simulink model "SimulacaoMaquinaCCBlocoConstruido"  (R2022b)
settings: Solver=VariableStepAuto  StartTime=0.0  StopTime=10  MaxStep=1e-4  RelTol=1e-3
libraries: spspowerguiLib x1
settings Model: Creator=marcone.faria  LastModifiedBy=dedep
settings ModelReferenceCC: EnableRefExpFcnMdlSchedulingChecks=on

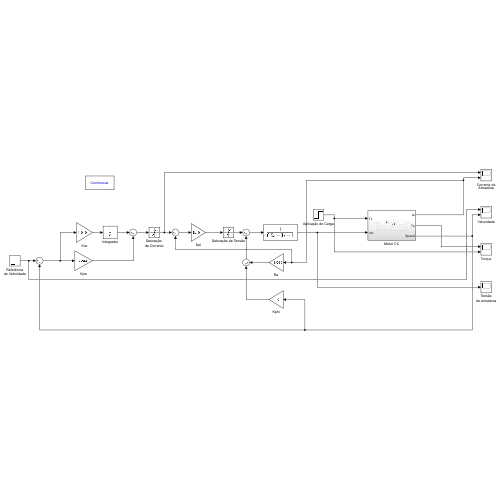
[thumbnail: Simulink's stored preview of the top-level diagram]
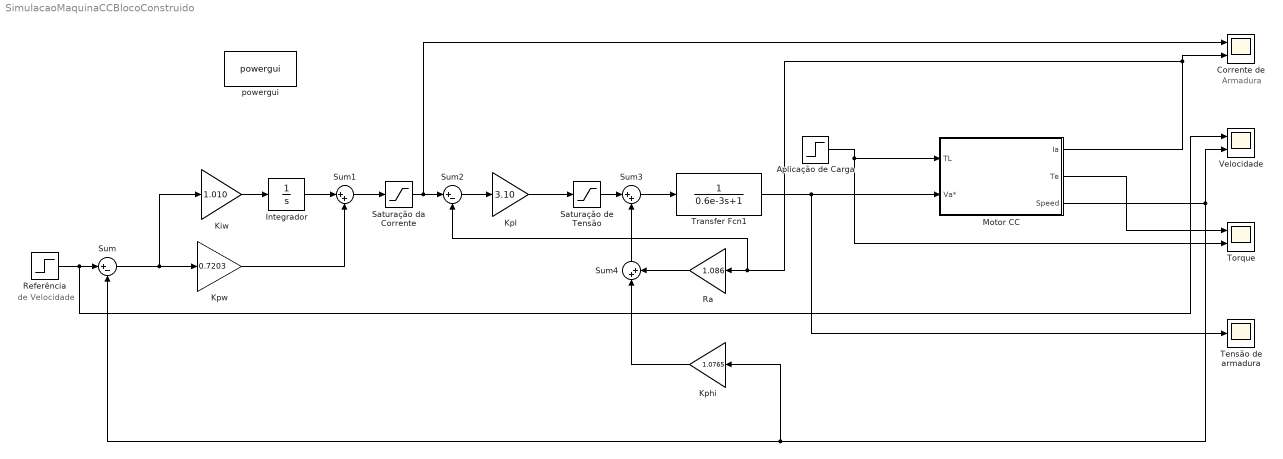
== system SimulacaoMaquinaCCBlocoConstruido ==
  note: Armadura
  note: de Velocidade
  Aplicação de Carga : Step  Before=20  After=40  SampleTime=0
  Corrente de : Scope  NumInputPorts=2
  Integrador : TransferFcn  Denominator=[1 0]
  Kiw : Gain  Gain=1.010
  Kphi : Gain  Gain=1.0765
  Kpl : Gain  Gain=3.10
  Kpw : Gain  Gain=0.7203
  Motor CC : Subsystem
  Ra : Gain  Gain=1.086
  Referência : Step  Time=0  After=92  SampleTime=0
  Saturação da Corrente : Saturate  UpperLimit=72  LowerLimit=-72
  Saturação de Tensão : Saturate  UpperLimit=360  LowerLimit=-360
  Sum : Sum  Inputs=|+-
  Sum1 : Sum  Inputs=|++
  Sum2 : Sum  Inputs=|+-
  Sum3 : Sum  Inputs=|++
  Sum4 : Sum  Inputs=|++
  Tensão de armadura : Scope
  Torque : Scope  NumInputPorts=2
  Transfer Fcn1 : TransferFcn  Denominator=[0.6e-3 1]
  Velocidade : Scope  NumInputPorts=2
  powergui : spspowerguiLib/powergui  Priority=1  SimulationMode=Continuous  SampleTime=50e-6  frequency=60  Iterations=50  frequencyindice=0  Pbase=100e6  ErrMax=1e-4  UnitsV=kV  UnitsW=MW  buscounter=0  FunctionMessages=off  echomessages=off  EnableUseOfTLC=off  CurrentSourceSwitches=off  DisableSnubberDevices=off  DisableRonSwitches=off  DisableVfSwitches=off  DisplayEquations=off  AutomaticDiscreteSolvers=off  SolverType=Tustin/Backward Euler (TBE)  Interpol=off  ExternalGateDelay=off  methode=off  Ts=100  x0status=blocks  SPID=on  SwTol=0  HookPort=off  NonlinearTolerance=1e-4  nMaxIteration=100  ContinueOnMaxIteration=off  RestoreLinks=warning  ResistiveCurrentMeasurement=off  Frange=[0:2:500]  Ylog=off  Xlog=on  ShowGrid=off  save=off  variable=ZData  structure=0  ZoomFFT=off  StartTime=0.0  cycles=1  DisplayStyle=1  fundamental=60  FreqAxis=off  MaxFrequency=1000  frequencyindicesteady=1  RmsSteady=1  display=off
  wires:
  Referência/1 -> Velocidade/1, Sum/1
  Sum/1 -> Kiw/1, Kpw/1
  Kiw/1 -> Integrador/1
  Integrador/1 -> Sum1/1
  Kpw/1 -> Sum1/2
  Sum1/1 -> Saturação da Corrente/1
  Saturação da Corrente/1 -> Corrente de/1, Sum2/1
  Sum2/1 -> Kpl/1
  Kpl/1 -> Saturação de Tensão/1
  Saturação de Tensão/1 -> Sum3/1
  Sum3/1 -> Transfer Fcn1/1
  Sum4/1 -> Sum3/2
  Ra/1 -> Sum4/2
  Kphi/1 -> Sum4/1
  Aplicação de Carga/1 -> Motor CC/1(TL), Torque/2
  Transfer Fcn1/1 -> Tensão de armadura/1, Motor CC/2(Va*)
  Motor CC/3(Speed) -> Velocidade/2, Kphi/1, Sum/2
  Motor CC/1(Ia) -> Corrente de/2, Sum2/2, Ra/1
  Motor CC/2(Te) -> Torque/1

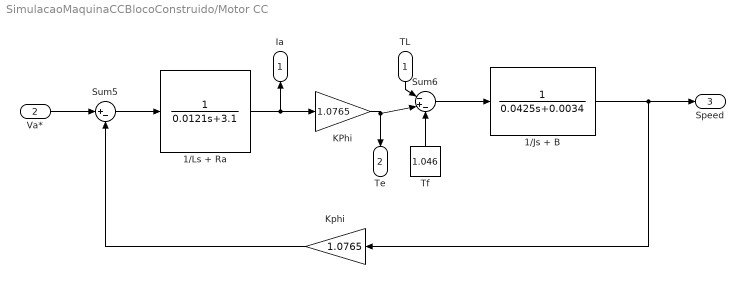
== system SimulacaoMaquinaCCBlocoConstruido/Motor CC ==
  TL : Inport
  Va* : Inport  Port=2
  1/Js + B : TransferFcn  Denominator=[0.0425 0.0034]
  1/Ls + Ra : TransferFcn  Denominator=[0.0121 3.1]
  KPhi : Gain  Gain=1.0765
  Kphi : Gain  Gain=1.0765
  Sum5 : Sum  Inputs=|+-
  Sum6 : Sum  Inputs=|-+-
  Tf : Constant  Value=1.046
  Ia : Outport
  Te : Outport  Port=2
  Speed : Outport  Port=3
  wires:
  1/Js + B/1 -> Kphi/1, Speed/1
  KPhi/1 -> Sum6/2, Te/1
  Tf/1 -> Sum6/3
  Sum5/1 -> 1/Ls + Ra/1
  1/Ls + Ra/1 -> KPhi/1, Ia/1
  Va*/1 -> Sum5/1
  Kphi/1 -> Sum5/2
  Sum6/1 -> 1/Js + B/1
  TL/1 -> Sum6/1
